simulink model "mainPacemakerUART"  (R2022b)
settings: Solver=FixedStepAuto  StartTime=0.0  StopTime=10.0  FixedStep=1e-3  RelTol=1e-3  EnableMultiTasking=on
undefined symbols (not defined in the file): A0, A1, D0, D1, D10, D11, D12, D13, D2, D3, D4, D5, D6, D7, D8, D9, PTA0, PTA1, PTA2, PTB2, PTB23, PTB3, PTB9, PTC16, PTC17, PTC2, PTC3, PTC4, PTD0, PTD1, PTD2, PTD3
libraries: frdmk64flib x19, etargetslib x10, simulink x2, dspstat3 x1
settings Model: ExtModeTrigDuration=5  Creator=christyjoseph-anton  LastModifiedBy=nickg
settings SolverCC: AlgebraicLoopSolver=TrustRegion
settings OptimizationCC: EnhancedBackFolding=on  PassReuseOutputArgsAs=Individual arguments  ZeroExternalMemoryAtStartup=off  ZeroInternalMemoryAtStartup=off  MaxStackSize=64  OptimizeBlockOrder=speed  DifferentSizesBufferReuse=on  OptimizationCustomize=off  EfficientTunableParamExpr=on
settings DebuggingCC: ParameterTunabilityLossMsg=error  UnconnectedInputMsg=warning  UnconnectedOutputMsg=warning  UnconnectedLineMsg=warning  SFMachineParentedDataDiag=warning
settings HardwareCC: ProdBitPerPointer=32  ProdBitPerSizeT=32  ProdBitPerPtrDiffT=32  ProdLargestAtomicInteger=Long  ProdLargestAtomicFloat=Double  ProdWordSize=32  ProdHWDeviceType=ARM Compatible->ARM Cortex
settings ModelReferenceCC: EnableRefExpFcnMdlSchedulingChecks=on
settings SFSimCC: MATLABDynamicMemAlloc=off
settings RTWCC: Description=Embedded Coder  SystemTargetFile=ert.tlc  HardwareBoard=NXP FRDM-K64F  TLCOptions="-aInlineSetEventsForThisBaseRateFcn=TLC_FALSE -aSuppressMultiTaskScheduler=TLC_FALSE  -aRateBasedStepFcn=0"  TemplateMakefile=ert_default_tmf  Toolchain=GNU Tools for ARM Embedded Processors  DLArmComputeVersion=19.05
settings CodeAppCC: ForceParamTrailComments=on  IgnoreCustomStorageClasses=off  OperatorAnnotations=on  SimulinkDataObjDesc=on  SFDataObjDesc=on  InsertBlockDesc=on
settings ERTTargetCC: ExtModeTransport=4  ExtModeMexFile=sendToCommService

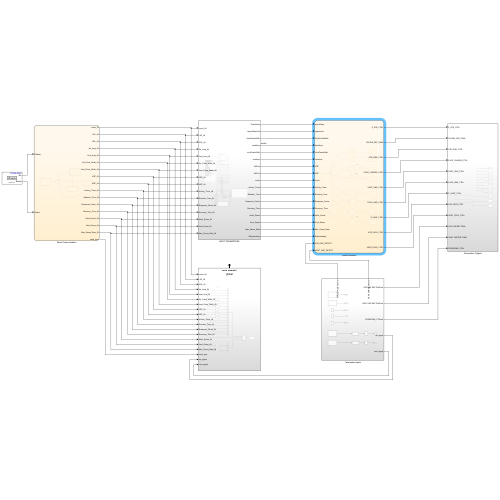
[thumbnail: Simulink's stored preview of the top-level diagram]
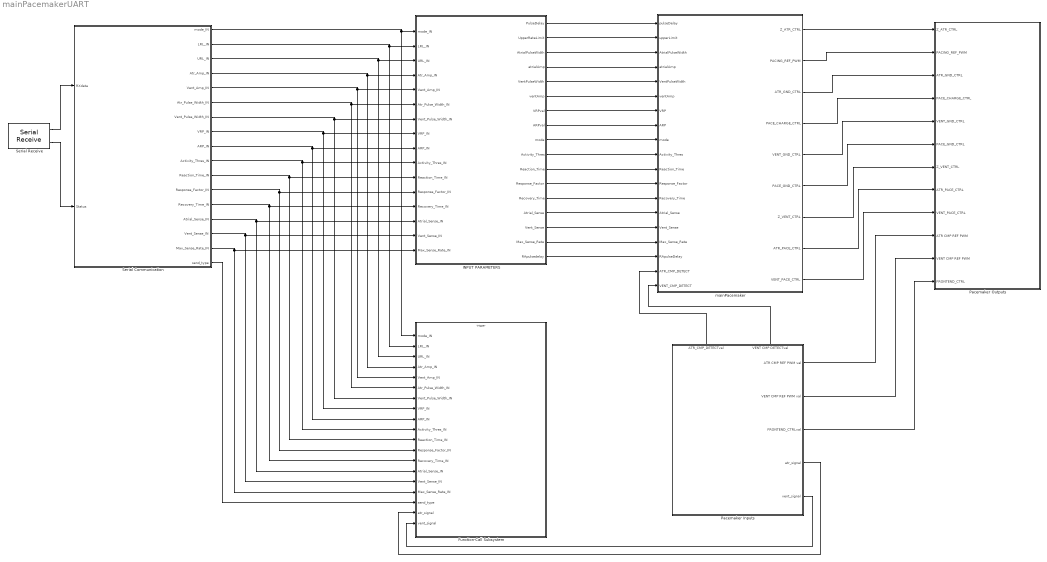
== system mainPacemakerUART ==
  Function-Call Subsystem : Subsystem  TreatAsAtomicUnit=on
  INPUT PARAMETERS : Subsystem
  Pacemaker Inputs : Subsystem
      settings: PortSchema="{\"entries\":[{\"content\":{\"sides\":[{\"content\":{\"connectorIds\":[]},\"type\":\"ConnectorPlacement.EquallySpacedRectSide\",\"uuid\":\"669aed97-6afe-41f5-9681-72417bc28ad7\"},{\"content\":{\"connectorIds\":[\"Out1\",\"Out2\",\"Out3\",\"Out4\",\"Out5\"],\"side\":\"RIGHT\"},\"type\":\"ConnectorPlacement.EquallySpacedRectSide\",\"uuid\":\"4d5229ba-5f7f-4491-b5d3-5b44c05a4562\"},{\"content\":{\"connectorIds\":[\"Out6\",\"Out7\"],\"side\":\"TOP\"},\"type\":\"ConnectorPlacement.EquallySpacedRectSide\",\"uuid\":\"a8fa4d81-6f15-4faa-ada6-82cdebea0c9a\"},{\"content\":{\"connectorIds\":[],\"side\":\"HIDDEN\"},\"type\":\"ConnectorPlacement.EquallySpacedRectSide\",\"uuid\":\"2be4ddd2-f58e-4c63-9a31-28b31fed5141\"}]},\"type\":\"ConnectorPlacement.EquallySpacedConnector\",\"uuid\":\"3d10de13-acf3-4b06-8558-a802ff7a980e\"}],\"packageUris\":[\"http://schema.mathworks.com/mf0/Connector/R2020b\"],\"version\":\"1.0\"}"
  Pacemaker Outputs : Subsystem
  Serial Communication : Stateflow chart  TreatAsAtomicUnit=on
      settings: PortSchema="{\"entries\":[{\"content\":{\"sides\":[{\"content\":{\"connectorIds\":[\"In1\",\"In2\"]},\"type\":\"ConnectorPlacement.EquallySpacedRectSide\",\"uuid\":\"155cda33-ed32-4503-9511-04db69497ed1\"},{\"content\":{\"connectorIds\":[\"Out1\",\"Out2\",\"Out3\",\"Out4\",\"Out5\",\"Out6\",\"Out7\",\"Out8\",\"Out9\",\"Out10\",\"Out11\",\"Out12\",\"Out13\",\"Out15\",\"Out16\",\"Out17\",\"Out14\"],\"side\":\"RIGHT\"},\"type\":\"ConnectorPlacement.EquallySpacedRectSide\",\"uuid\":\"03ebeb28-7a83-492d-8c6c-4e2462ffa620\"},{\"content\":{\"connectorIds\":[],\"side\":\"TOP\"},\"type\":\"ConnectorPlacement.EquallySpacedRectSide\",\"uuid\":\"df4d072d-cc91-443f-87bb-f397160e1321\"},{\"content\":{\"connectorIds\":[],\"side\":\"HIDDEN\"},\"type\":\"ConnectorPlacement.EquallySpacedRectSide\",\"uuid\":\"7e82692c-c04b-4422-948f-81d628cdafb4\"}]},\"type\":\"ConnectorPlacement.EquallySpacedConnector\",\"uuid\":\"d94360bd-ed44-4ec4-9498-3e1b8fe58b8b\"}],\"packageUris\":[\"http://schema.mathworks.com/mf0/Connector/R2020b\"],\"version\":\"1.0\"}"
  Serial Receive : frdmk64flib/Serial Receive  SCIModule=0  Baudrate=uint32(9600)  Parity=None  StopBits=1  HardwareFlowControl=None  ByteOrder=LittleEndian  DataType=uint8  DataLength=74  BlockingMode=off  OutputStatus=on  SampleTime=-1
  mainPacemaker : Stateflow chart  TreatAsAtomicUnit=on
      settings: PortSchema="{\"entries\":[{\"content\":{\"sides\":[{\"content\":{\"connectorIds\":[\"In1\",\"In2\",\"In3\",\"In4\",\"In6\",\"In7\",\"In8\",\"In9\",\"In5\",\"In10\",\"In11\",\"In12\",\"In13\",\"In14\",\"In15\",\"In18\",\"In17\",\"In16\",\"In19\"]},\"type\":\"ConnectorPlacement.EquallySpacedRectSide\",\"uuid\":\"201ff05f-9430-4aaf-95e3-1c7ad2916a7e\"},{\"content\":{\"connectorIds\":[\"Out1\",\"Out2\",\"Out3\",\"Out4\",\"Out5\",\"Out6\",\"Out7\",\"Out8\",\"Out9\"],\"side\":\"RIGHT\"},\"type\":\"ConnectorPlacement.EquallySpacedRectSide\",\"uuid\":\"5d74b1aa-6a43-4298-b365-ae775337f59f\"},{\"content\":{\"connectorIds\":[],\"side\":\"TOP\"},\"type\":\"ConnectorPlacement.EquallySpacedRectSide\",\"uuid\":\"2dd794d3-9ac6-4b1a-b21d-1675ed402b7f\"},{\"content\":{\"connectorIds\":[],\"side\":\"HIDDEN\"},\"type\":\"ConnectorPlacement.EquallySpacedRectSide\",\"uuid\":\"1f2ef5a6-ce50-482f-afd9-c477b13c6922\"}]},\"type\":\"ConnectorPlacement.EquallySpacedConnector\",\"uuid\":\"6e887b8a-81a7-4209-ac77-3100cf09278d\"}],\"packageUris\":[\"http://schema.mathworks.com/mf0/Connector/R2020b\"],\"version\":\"1.0\"}"
  wires:
  INPUT PARAMETERS/3(AtrialPulseWidth) -> mainPacemaker/3(AtrialPulseWidth)
  INPUT PARAMETERS/4(atrialAmp) -> mainPacemaker/4(atrialAmp)
  INPUT PARAMETERS/1(PulseDelay) -> mainPacemaker/1(pulseDelay)
  INPUT PARAMETERS/2(UpperRateLimit) -> mainPacemaker/2(upperLimit)
  INPUT PARAMETERS/5(VentPulseWidth) -> mainPacemaker/6(VentPulseWidth)
  INPUT PARAMETERS/6(ventAmp) -> mainPacemaker/7(ventAmp)
  INPUT PARAMETERS/7(VRPval) -> mainPacemaker/8(VRP)
  INPUT PARAMETERS/8(ARPval) -> mainPacemaker/9(ARP)
  Pacemaker Inputs/6(ATR_CMP_DETECTval) -> mainPacemaker/16(ATR_CMP_DETECT)
  Pacemaker Inputs/7(VENT CMP DETECTval) -> mainPacemaker/19(VENT_CMP_DETECT)
  mainPacemaker/1(Z_ATR_CTRL) -> Pacemaker Outputs/1(Z_ATR_CTRL)
  mainPacemaker/2(PACING_REF_PWM) -> Pacemaker Outputs/2(PACING_REF_PWM)
  mainPacemaker/3(ATR_GND_CTRL) -> Pacemaker Outputs/3(ATR_GND_CTRL)
  mainPacemaker/4(PACE_CHARGE_CTRL) -> Pacemaker Outputs/4(PACE_CHARGE_CTRL)
  mainPacemaker/5(VENT_GND_CTRL) -> Pacemaker Outputs/5(VENT_GND_CTRL)
  mainPacemaker/6(PACE_GND_CTRL) -> Pacemaker Outputs/6(PACE_GND_CTRL)
  mainPacemaker/7(Z_VENT_CTRL) -> Pacemaker Outputs/7(Z_VENT_CTRL)
  mainPacemaker/8(ATR_PACE_CTRL) -> Pacemaker Outputs/8(ATR_PACE_CTRL)
  mainPacemaker/9(VENT_PACE_CTRL) -> Pacemaker Outputs/9(VENT_PACE_CTRL)
  Pacemaker Inputs/1(ATR CMP REF PWM val) -> Pacemaker Outputs/10(ATR CMP REF PWM)
  Pacemaker Inputs/2(VENT CMP REF PWM val) -> Pacemaker Outputs/11(VENT CMP REF PWM)
  Pacemaker Inputs/3(FRONTEND_CTRLval) -> Pacemaker Outputs/12(FRONTEND_CTRL)
  INPUT PARAMETERS/9(mode) -> mainPacemaker/5(mode)
  Serial Communication/1(mode_IN) -> Function-Call Subsystem/1(mode_IN), INPUT PARAMETERS/1(mode_IN)
  Serial Communication/2(LRL_IN) -> Function-Call Subsystem/2(LRL_IN), INPUT PARAMETERS/2(LRL_IN)
  Serial Communication/3(URL_IN) -> Function-Call Subsystem/3(URL_IN), INPUT PARAMETERS/3(URL_IN)
  Serial Communication/4(Atr_Amp_IN) -> Function-Call Subsystem/4(Atr_Amp_IN), INPUT PARAMETERS/4(Atr_Amp_IN)
  Serial Communication/5(Vent_Amp_IN) -> Function-Call Subsystem/5(Vent_Amp_IN), INPUT PARAMETERS/5(Vent_Amp_IN)
  Serial Communication/6(Atr_Pulse_Width_IN) -> Function-Call Subsystem/6(Atr_Pulse_Width_IN), INPUT PARAMETERS/6(Atr_Pulse_Width_IN)
  Serial Communication/7(Vent_Pulse_Width_IN) -> Function-Call Subsystem/7(Vent_Pulse_Width_IN), INPUT PARAMETERS/7(Vent_Pulse_Width_IN)
  Serial Communication/8(VRP_IN) -> Function-Call Subsystem/8(VRP_IN), INPUT PARAMETERS/8(VRP_IN)
  Serial Communication/9(ARP_IN) -> Function-Call Subsystem/9(ARP_IN), INPUT PARAMETERS/9(ARP_IN)
  Serial Receive/2 -> Serial Communication/2(Status)
  Serial Receive/1 -> Serial Communication/1(RXdata)
  Serial Communication/10(Activity_Thres_IN) -> INPUT PARAMETERS/10(Activity_Thres_IN), Function-Call Subsystem/10(Activity_Thres_IN)
  Serial Communication/11(Reaction_Time_IN) -> Function-Call Subsystem/11(Reaction_Time_IN), INPUT PARAMETERS/11(Reaction_Time_IN)
  Serial Communication/12(Response_Factor_IN) -> Function-Call Subsystem/12(Response_Factor_IN), INPUT PARAMETERS/12(Response_Factor_IN)
  Serial Communication/13(Recovery_Time_IN) -> Function-Call Subsystem/13(Recovery_Time_IN), INPUT PARAMETERS/13(Recovery_Time_IN)
  INPUT PARAMETERS/10(Activity_Thres) -> mainPacemaker/10(Activity_Thres)
  INPUT PARAMETERS/11(Reaction_Time) -> mainPacemaker/11(Reaction_Time)
  INPUT PARAMETERS/12(Response_Factor) -> mainPacemaker/12(Response_Factor)
  INPUT PARAMETERS/13(Recovery_Time) -> mainPacemaker/13(Recovery_Time)
  Serial Communication/14(send_type) -> Function-Call Subsystem/17(send_type)
  Pacemaker Inputs/4(atr_signal) -> Function-Call Subsystem/18(atr_signal)
  Pacemaker Inputs/5(vent_signal) -> Function-Call Subsystem/19(vent_signal)
  INPUT PARAMETERS/14(Atrial_Sense) -> mainPacemaker/14(Atrial_Sense)
  INPUT PARAMETERS/15(Vent_Sense) -> mainPacemaker/15(Vent_Sense)
  INPUT PARAMETERS/16(Max_Sense_Rate) -> mainPacemaker/18(Max_Sense_Rate)
  Serial Communication/15(Atrial_Sense_IN) -> INPUT PARAMETERS/14(Atrial_Sense_IN), Function-Call Subsystem/14(Atrial_Sense_IN)
  Serial Communication/16(Vent_Sense_IN) -> INPUT PARAMETERS/15(Vent_Sense_IN), Function-Call Subsystem/15(Vent_Sense_IN)
  Serial Communication/17(Max_Sense_Rate_IN) -> INPUT PARAMETERS/16(Max_Sense_Rate_IN), Function-Call Subsystem/16(Max_Sense_Rate_IN)
  INPUT PARAMETERS/17(RApulsedelay) -> mainPacemaker/17(RApulseDelay)

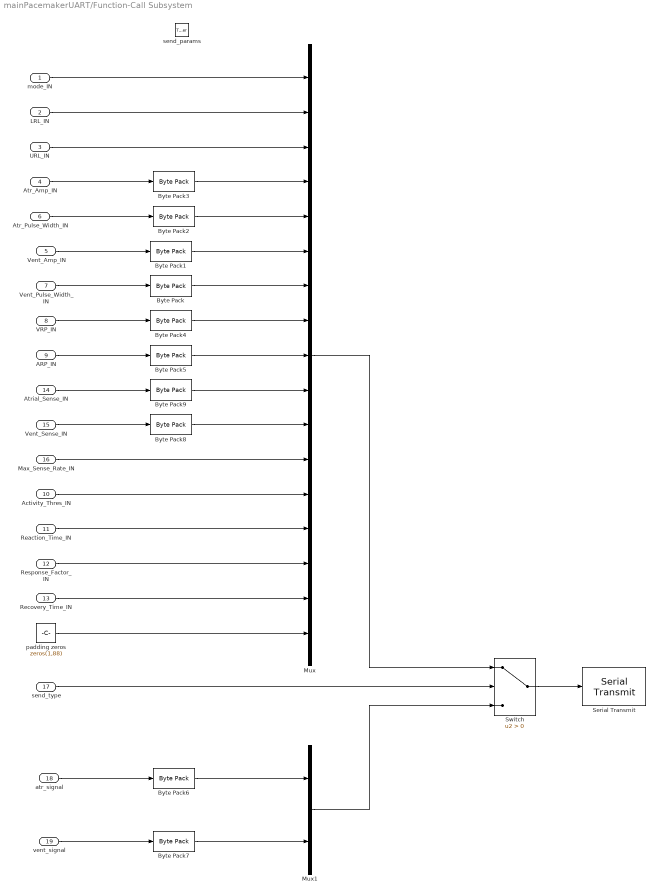
== system mainPacemakerUART/Function-Call Subsystem ==
  mode_IN : Inport
  LRL_IN : Inport  Port=2
  URL_IN : Inport  Port=3
  Atr_Amp_IN : Inport  Port=4
  Vent_Amp_IN : Inport  Port=5
  Atr_Pulse_Width_IN : Inport  Port=6
  Vent_Pulse_Width_IN : Inport  Port=7
  VRP_IN : Inport  Port=8
  ARP_IN : Inport  Port=9
  Activity_Thres_IN : Inport  Port=10
  Reaction_Time_IN : Inport  Port=11
  Response_Factor_IN : Inport  Port=12
  Recovery_Time_IN : Inport  Port=13
  Atrial_Sense_IN : Inport  Port=14
  Vent_Sense_IN : Inport  Port=15
  Max_Sense_Rate_IN : Inport  Port=16
  send_type : Inport  Port=17
  atr_signal : Inport  Port=18
  vent_signal : Inport  Port=19
  send_params : TriggerPort  TriggerType=function-call  IsSimulinkFunction=on  FunctionName=send_params  VariantControl=Variant
  Byte Pack{,1..9} (10 alike) : etargetslib/Byte Pack  datatypes={'double'}  byteAlign=1
  Mux : Mux  Inputs=17
  Mux1 : Mux  Inputs=2
  Serial Transmit : frdmk64flib/Serial Transmit  SCIModule=0  Baudrate=uint32(9600)  Parity=None  StopBits=1  HardwareFlowControl=None  ByteOrder=LittleEndian  BlockingMode=on  OutputStatus=off
  Switch : Switch  Criteria=u2 > Threshold  SaturateOnIntegerOverflow=off  InputSameDT=off
  padding zeros : Constant  Value=zeros(1,88)  OutDataTypeStr=uint8
  wires:
  mode_IN/1 -> Mux/1
  LRL_IN/1 -> Mux/2
  URL_IN/1 -> Mux/3
  Atr_Amp_IN/1 -> Byte Pack3/1
  Atr_Pulse_Width_IN/1 -> Byte Pack2/1
  Vent_Amp_IN/1 -> Byte Pack1/1
  Vent_Pulse_Width_IN/1 -> Byte Pack/1
  VRP_IN/1 -> Byte Pack4/1
  ARP_IN/1 -> Byte Pack5/1
  Byte Pack/1 -> Mux/7
  Byte Pack1/1 -> Mux/6
  Byte Pack3/1 -> Mux/4
  Byte Pack2/1 -> Mux/5
  Byte Pack4/1 -> Mux/8
  Byte Pack5/1 -> Mux/9
  Switch/1 -> Serial Transmit/1
  Mux/1 -> Switch/1
  send_type/1 -> Switch/2
  Mux1/1 -> Switch/3
  atr_signal/1 -> Byte Pack6/1
  Byte Pack6/1 -> Mux1/1
  vent_signal/1 -> Byte Pack7/1
  Byte Pack7/1 -> Mux1/2
  padding zeros/1 -> Mux/17
  Atrial_Sense_IN/1 -> Byte Pack9/1
  Vent_Sense_IN/1 -> Byte Pack8/1
  Activity_Thres_IN/1 -> Mux/13
  Reaction_Time_IN/1 -> Mux/14
  Response_Factor_IN/1 -> Mux/15
  Recovery_Time_IN/1 -> Mux/16
  Byte Pack8/1 -> Mux/11
  Max_Sense_Rate_IN/1 -> Mux/12
  Byte Pack9/1 -> Mux/10

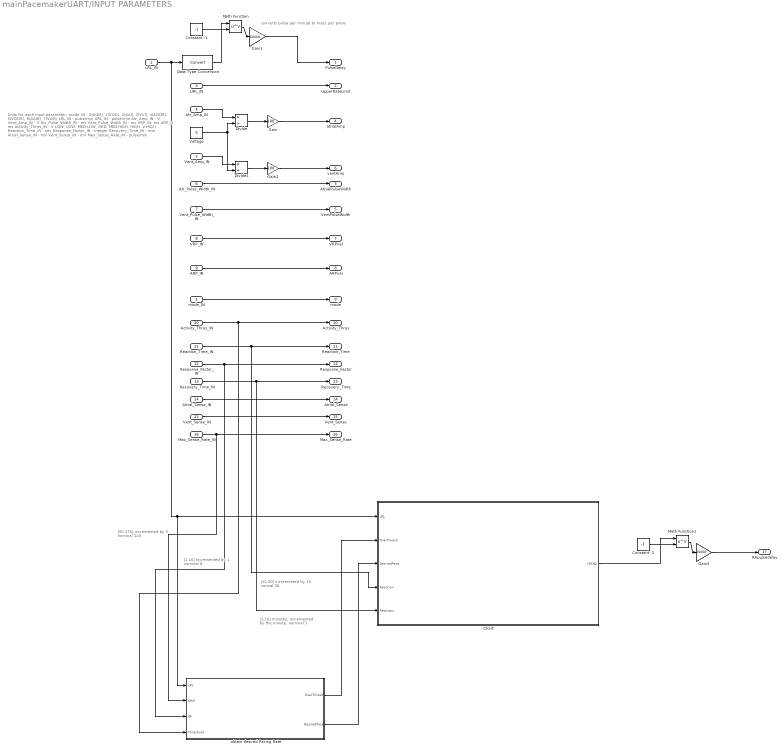
== system mainPacemakerUART/INPUT PARAMETERS ==
  note: Units for each input parameter:
      | mode_IN - 0(AOO), 1(VOO), 2(AAI), 3(VVI), 4(AOOR), 5(VOOR), 6(AAIR), 7(VVIR)
      |
      | LRL_IN - pulse/min
      |
      | URL_IN - pulse/min
      |
      | Atr_Amp_IN - V
      |
      | Vent_Amp_IN - V
      |
      | Atr_Pulse_Width_IN - ms
      |
      | Vent_Pulse_Width_IN - ms
      |
      | VRP_IN- ms ARP_N - ms
      |
      | Activity_Thres_IN - V-LOW, LOW, MED-LOW, MED, MED-HIGH, HIGH, V-HIGH
      |
      | Reaction_Time_IN - sec
      |
      | Response_Factor_IN - integer
      |
      | Recovery_Time_IN - min Atrial_Sense_IN - mV
      |
      | Vent_Sense_IN - mV
      |
      | Max_Sense_Rate_IN - pulse/min
  note: converts pulse per minute to msec per pulse
  note: [2,16] minutes, incremented by the minute, nominal 5
  note: [10,50] incremented by 10 nomial 30
  note: [50,175] incremented by 5 nominal 120
  note: [1,16] incremented by 1, nominal 8
  mode_IN : Inport
  LRL_IN : Inport  Port=2
  URL_IN : Inport  Port=3
  Atr_Amp_IN : Inport  Port=4
  Vent_Amp_IN : Inport  Port=5
  Atr_Pulse_Width_IN : Inport  Port=6
  Vent_Pulse_Width_IN : Inport  Port=7
  VRP_IN : Inport  Port=8
  ARP_IN : Inport  Port=9
  Activity_Thres_IN : Inport  Port=10
  Reaction_Time_IN : Inport  Port=11
  Response_Factor_IN : Inport  Port=12
  Recovery_Time_IN : Inport  Port=13
  Atrial_Sense_IN : Inport  Port=14
  Vent_Sense_IN : Inport  Port=15
  Max_Sense_Rate_IN : Inport  Port=16
  Chart : Stateflow chart  TreatAsAtomicUnit=on
  Constant -1 : Constant  Value=-1
  Constant -2 : Constant  Value=-1
  Data Type Conversion : DataTypeConversion  SaturateOnIntegerOverflow=off  RndMeth=Floor
  Divide : Product  Inputs=*/
  Divide1 : Product  Inputs=*/
  Gain : Gain  Gain=100
  Gain1 : Gain  Gain=60000
  Gain2 : Gain  Gain=100
  Gain3 : Gain  Gain=60000
  Math Function : Math  Operator=pow
  Math Function1 : Math  Operator=pow
  Voltage : Constant  Value=5
  obtain desired Pacing Rate : Subsystem
  PulseDelay : Outport
  UpperRateLimit : Outport  Port=2
  AtrialPulseWidth : Outport  Port=3
  atrialAmp : Outport  Port=4  OutDataTypeStr=double
  VentPulseWidth : Outport  Port=5
  ventAmp : Outport  Port=6
  VRPval : Outport  Port=7
  ARPval : Outport  Port=8
  mode : Outport  Port=9
  Activity_Thres : Outport  Port=10
  Reaction_Time : Outport  Port=11
  Response_Factor : Outport  Port=12
  Recovery_Time : Outport  Port=13
  Atrial_Sense : Outport  Port=14
  Vent_Sense : Outport  Port=15
  Max_Sense_Rate : Outport  Port=16
  RApulsedelay : Outport  Port=17
  wires:
  Gain/1 -> atrialAmp/1
  Constant -1/1 -> Math Function/2
  Math Function/1 -> Gain1/1
  Atr_Amp_IN/1 -> Divide/1
  Gain1/1 -> PulseDelay/1
  URL_IN/1 -> UpperRateLimit/1
  Atr_Pulse_Width_IN/1 -> AtrialPulseWidth/1
  Divide/1 -> Gain/1
  Voltage/1 -> Divide1/2, Divide/2
  Gain2/1 -> ventAmp/1
  Vent_Amp_IN/1 -> Divide1/1
  Divide1/1 -> Gain2/1
  Vent_Pulse_Width_IN/1 -> VentPulseWidth/1
  VRP_IN/1 -> VRPval/1
  ARP_IN/1 -> ARPval/1
  mode_IN/1 -> mode/1
  Data Type Conversion/1 -> Math Function/1
  Vent_Sense_IN/1 -> Vent_Sense/1
  Atrial_Sense_IN/1 -> Atrial_Sense/1
  Recovery_Time_IN/1 -> Chart/5(Recovery), Recovery_Time/1
  Activity_Thres_IN/1 -> obtain desired Pacing Rate/4(Threshold), Activity_Thres/1
  Reaction_Time_IN/1 -> Chart/4(Reaction), Reaction_Time/1
  obtain desired Pacing Rate/2(DesiredPace) -> Chart/3(DesiredPace)
  obtain desired Pacing Rate/1(OverThresh) -> Chart/2(OverThresh)
  Response_Factor_IN/1 -> Response_Factor/1, obtain desired Pacing Rate/3(RF)
  LRL_IN/1 -> Chart/1(LRL), obtain desired Pacing Rate/1(LRL), Data Type Conversion/1
  Max_Sense_Rate_IN/1 -> obtain desired Pacing Rate/2(MSR), Max_Sense_Rate/1
  Math Function1/1 -> Gain3/1
  Chart/1(LRLRA) -> Math Function1/1
  Constant -2/1 -> Math Function1/2
  Gain3/1 -> RApulsedelay/1

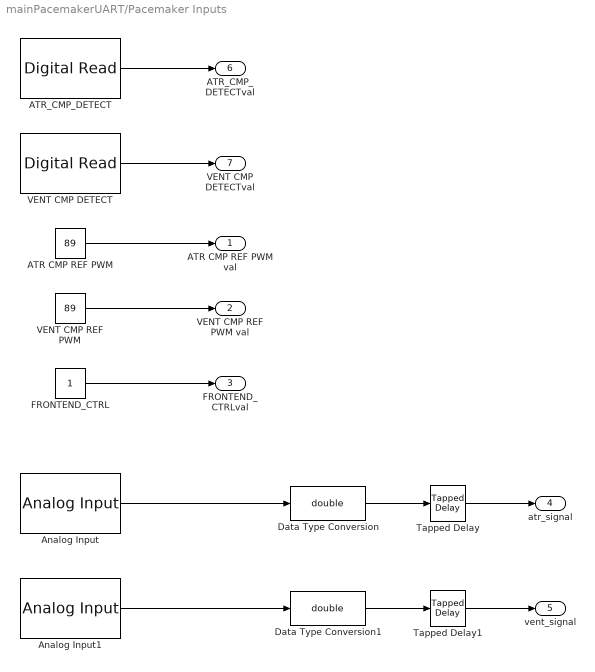
== system mainPacemakerUART/Pacemaker Inputs ==
  ATR CMP REF PWM : Constant  Value=89
  ATR_CMP_DETECT : frdmk64flib/Digital Read  Whichpin=PTC16 (D0)  SampleTime=-1
  Analog Input : frdmk64flib/Analog Input  Whichpin=PTB2 (A0)  SampleTime=-1
  Analog Input1 : frdmk64flib/Analog Input  Whichpin=PTB3 (A1)  SampleTime=-1
  Data Type Conversion : DataTypeConversion  OutDataTypeStr=double  SaturateOnIntegerOverflow=off  RndMeth=Floor
  Data Type Conversion1 : DataTypeConversion  OutDataTypeStr=double  SaturateOnIntegerOverflow=off  RndMeth=Floor
  FRONTEND_CTRL : Constant
  Tapped Delay : simulink/Discrete/Tapped Delay  vinit=1  samptime=0.002  NumDelays=10  DelayOrder=Oldest  includeCurrent=off
  Tapped Delay1 : simulink/Discrete/Tapped Delay  vinit=0.0  samptime=0.002  NumDelays=10  DelayOrder=Oldest  includeCurrent=off
  VENT CMP DETECT : frdmk64flib/Digital Read  Whichpin=PTC17 (D1)  SampleTime=-1
  VENT CMP REF PWM : Constant  Value=89
  ATR CMP REF PWM val : Outport
  VENT CMP REF PWM val : Outport  Port=2
  FRONTEND_CTRLval : Outport  Port=3
  atr_signal : Outport  Port=4
  vent_signal : Outport  Port=5
  ATR_CMP_DETECTval : Outport  Port=6
  VENT CMP DETECTval : Outport  Port=7
  wires:
  VENT CMP DETECT/1 -> VENT CMP DETECTval/1
  VENT CMP REF PWM/1 -> VENT CMP REF PWM val/1
  ATR_CMP_DETECT/1 -> ATR_CMP_DETECTval/1
  ATR CMP REF PWM/1 -> ATR CMP REF PWM val/1
  FRONTEND_CTRL/1 -> FRONTEND_CTRLval/1
  Analog Input/1 -> Data Type Conversion/1
  Data Type Conversion/1 -> Tapped Delay/1
  Analog Input1/1 -> Data Type Conversion1/1
  Data Type Conversion1/1 -> Tapped Delay1/1
  Tapped Delay/1 -> atr_signal/1
  Tapped Delay1/1 -> vent_signal/1

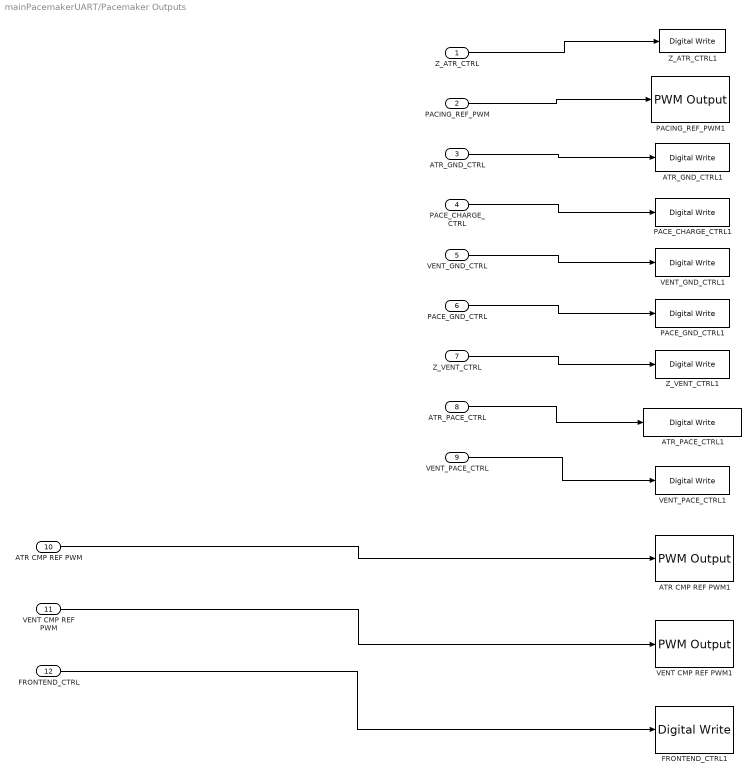
== system mainPacemakerUART/Pacemaker Outputs ==
  Z_ATR_CTRL : Inport
  PACING_REF_PWM : Inport  Port=2
  ATR_GND_CTRL : Inport  Port=3
  PACE_CHARGE_CTRL : Inport  Port=4
  VENT_GND_CTRL : Inport  Port=5
  PACE_GND_CTRL : Inport  Port=6
  Z_VENT_CTRL : Inport  Port=7
  ATR_PACE_CTRL : Inport  Port=8
  VENT_PACE_CTRL : Inport  Port=9
  ATR CMP REF PWM : Inport  Port=10
  VENT CMP REF PWM : Inport  Port=11
  FRONTEND_CTRL : Inport  Port=12
  ATR CMP REF PWM1 : frdmk64flib/PWM Output  Whichpin=PTC2 (D6)  InitialFrequency=2000  InitialDutyCycle=0
  ATR_GND_CTRL1 : frdmk64flib/Digital Write  Whichpin=PTD2 (D11)
  ATR_PACE_CTRL1 : frdmk64flib/Digital Write  Whichpin=PTA0 (D8)
  FRONTEND_CTRL1 : frdmk64flib/Digital Write  Whichpin=PTD1 (D13)
  PACE_CHARGE_CTRL1 : frdmk64flib/Digital Write  Whichpin=PTB9 (D2)
  PACE_GND_CTRL1 : frdmk64flib/Digital Write  Whichpin=PTD0 (D10)
  PACING_REF_PWM1 : frdmk64flib/PWM Output  Whichpin=PTA2 (D5)  InitialFrequency=2000  InitialDutyCycle=50
  VENT CMP REF PWM1 : frdmk64flib/PWM Output  Whichpin=PTA1 (D3)  InitialFrequency=2000  InitialDutyCycle=0
  VENT_GND_CTRL1 : frdmk64flib/Digital Write  Whichpin=PTD3 (D12)
  VENT_PACE_CTRL1 : frdmk64flib/Digital Write  Whichpin=PTC4 (D9)
  Z_ATR_CTRL1 : frdmk64flib/Digital Write  Whichpin=PTB23 (D4)
  "Z_VENT_CTRL1 " : frdmk64flib/Digital Write  Whichpin=PTC3 (D7)
  wires:
  ATR_PACE_CTRL/1 -> ATR_PACE_CTRL1/1
  ATR CMP REF PWM/1 -> ATR CMP REF PWM1/1
  PACING_REF_PWM/1 -> PACING_REF_PWM1/1
  VENT_GND_CTRL/1 -> VENT_GND_CTRL1/1
  VENT CMP REF PWM/1 -> VENT CMP REF PWM1/1
  VENT_PACE_CTRL/1 -> VENT_PACE_CTRL1/1
  PACE_CHARGE_CTRL/1 -> PACE_CHARGE_CTRL1/1
  Z_VENT_CTRL/1 -> "Z_VENT_CTRL1 "/1
  Z_ATR_CTRL/1 -> Z_ATR_CTRL1/1
  ATR_GND_CTRL/1 -> ATR_GND_CTRL1/1
  FRONTEND_CTRL/1 -> FRONTEND_CTRL1/1
  PACE_GND_CTRL/1 -> PACE_GND_CTRL1/1

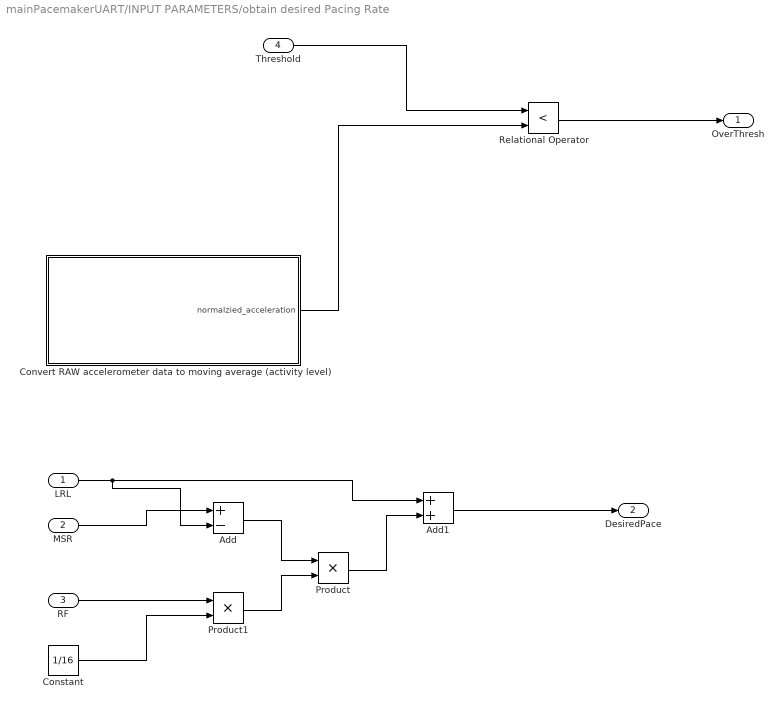
== system mainPacemakerUART/INPUT PARAMETERS/obtain desired Pacing Rate ==
  LRL : Inport
  MSR : Inport  Port=2
  RF : Inport  Port=3
  Threshold : Inport  Port=4
  Add : Sum  Inputs=+-
  Add1 : Sum
  Constant : Constant  Value=1/16
  Convert RAW accelerometer data to moving average (activity level) : Subsystem
  Product : Product
  Product1 : Product
  Relational Operator : RelationalOperator  Operator=<  OutDataTypeStr=boolean  RndMeth=Simplest  InputSameDT=off
  OverThresh : Outport
  DesiredPace : Outport  Port=2
  wires:
  MSR/1 -> Add/1
  LRL/1 -> Add/2, Add1/1
  Add/1 -> Product/1
  Product/1 -> Add1/2
  Threshold/1 -> Relational Operator/1
  Add1/1 -> DesiredPace/1
  Relational Operator/1 -> OverThresh/1
  Convert RAW accelerometer data to moving average (activity level)/1(normalzied_acceleration) -> Relational Operator/2
  RF/1 -> Product1/1
  Constant/1 -> Product1/2
  Product1/1 -> Product/2

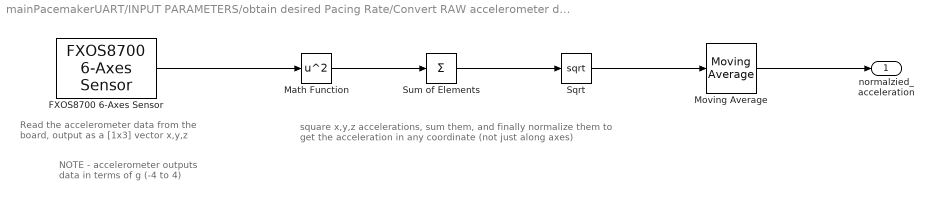
== system mainPacemakerUART/INPUT PARAMETERS/obtain desired Pacing Rate/Convert RAW accelerometer data to moving average (activity level) ==
  note: NOTE - accelerometer outputs data in terms of g (-4 to 4)
  note: square x,y,z accelerations, sum them, and finally normalize them to get the acceleration in any coordinate (not just along axes)
  note: Read the accelerometer data from the board, output as a [1x3] vector x,y,z
  FXOS8700 6-Axes Sensor : frdmk64flib/FXOS8700 6-Axes Sensor  Activesensor=Accelerometer only  ODR=800Hz  HybridODR=400Hz  Accelfullrange=-4g to +4g  SampleTime=-1
  Math Function : Math  Operator=square
  Moving Average : dspstat3/Moving Average  Method=Sliding window  ForgettingFactorPort=off  SpecifyWindowLength=on  WindowLength=4  OverlapLength=3  AllowArbitraryInputLength=off  ForgettingFactor=0.9  SimulateUsing=Code generation
  Sqrt : Sqrt
  Sum of Elements : Sum  Inputs=+
  normalzied_acceleration : Outport
  wires:
  Sum of Elements/1 -> Sqrt/1
  Sqrt/1 -> Moving Average/1
  Moving Average/1 -> normalzied_acceleration/1
  FXOS8700 6-Axes Sensor/1 -> Math Function/1
  Math Function/1 -> Sum of Elements/1

== stateflow chart mainPacemakerUART/Serial Communication ==
  settings: executeAtInitialization=1
  state SET_PARM
    entry:
    mode_IN=RXdata(3); %1B
    LRL_IN=RXdata(4); %1B
    URL_IN=RXdata(5); %1B
    Atr_Amp_IN=typecast(RXdata(6:13),'double'); %8B
    Atr_Pulse_Width_IN=typecast(RXdata(14:21),'double'); %8B
    Vent_Amp_IN=typecast(RXdata(22:29),'double') %8B
    Vent_Pulse_Width_IN=typecast(RXdata(30:37),'double'); %8B
    VRP_IN=typecast(RXdata(38:45),'double'); %8B
    ARP_IN=typecast(RXdata(46:53),'double'); %8B
    Atrial_Sense_IN=typecast(RXdata(54:61),'double'); %8B
    Vent_Sense_IN=typecast(RXdata(62:69),'double'); %8B
    Max_Sense_Rate_IN=RXdata(70); %1B
    Activity_Thres_IN=RXdata(71); %1B
    Reaction_Time_IN=RXdata(72); %1B
    Response_Factor_IN=RXdata(73); %1B
    Recovery_Time_IN=RXdata(74); %1B
  state setDefault
    entry:
    mode_IN = 3;
    LRL_IN = 60;
    URL_IN = 120;
    Atr_Amp_IN = 3.3;
    Vent_Amp_IN = 3.3;
    Atr_Pulse_Width_IN = 20;
    Vent_Pulse_Width_IN = 20;
    VRP_IN=320;
    ARP_IN=250;
    Activity_Thres_IN=3;
    Reaction_Time_IN=30;
    Response_Factor_IN=8;
    Recovery_Time_IN=5;
    Atrial_Sense_IN=0.75;
    Vent_Sense_IN=2.5;
    Max_Sense_Rate_IN=120;
  state STANDBY
    %Waiting for COM
  state ECHO_PARAM
    entry:
    send_type=1; %signals send block to echo parameters
    send_params();
  state ECG_SEND
    entry:
    send_type=0; %signals send block to send  ECG data
    send_params();
  SET_PARM -> STANDBY
  (junction 11) -> SET_PARM [order 1] : [RXdata(2)==hex2dec('55')]
  (default) -> setDefault
  (junction 8) -> STANDBY [order 2]
  setDefault -> STANDBY
  STANDBY -> (junction 8) : [Status==0]
  (junction 8) -> (junction 11) [order 1] : [RXdata(1)==hex2dec('16')]
  (junction 11) -> ECHO_PARAM [order 2] : [RXdata(2)==hex2dec('22')]
  (junction 11) -> ECG_SEND [order 3] : [RXdata(2)==hex2dec('77')]
  ECHO_PARAM -> STANDBY
  ECG_SEND -> STANDBY
  data: RXdata input uint8; Status input uint8; mode_IN output uint8; LRL_IN output uint8; URL_IN output uint8; Atr_Amp_IN output double; Vent_Amp_IN output double; Atr_Pulse_Width_IN output double; Vent_Pulse_Width_IN output double; VRP_IN output double; ARP_IN output double; Activity_Thres_IN output uint8; Reaction_Time_IN output uint8; Response_Factor_IN output uint8; Recovery_Time_IN output uint8; send_type output uint8; Atrial_Sense_IN output double; Vent_Sense_IN output double; Max_Sense_Rate_IN output uint8

== stateflow chart mainPacemakerUART/INPUT PARAMETERS/Chart ==
  state IncreaseRate
    LRLRA = LRLRA + ((double(DesiredPace) - double(LRL)) / double(Reaction)) / (1000)
  state S1
    LRLRA = double(LRL)
  state HoldDesiredPace
    LRLRA = double(DesiredPace)
  state ActivityBroken [commented out]
  state DecreaseRate
    LRLRA = LRLRA - ((double(DesiredPace) - double(LRL)) / double(Recovery)) / (1000)
  IncreaseRate -> HoldDesiredPace : [LRLRA >= DesiredPace]
  S1 -> IncreaseRate : [OverThresh == 1]
  DecreaseRate -> IncreaseRate [commented out] : [OverThresh == 1]
  IncreaseRate -> ActivityBroken [commented out] : [OverThresh ~= 1]
  ActivityBroken -> IncreaseRate [commented out] : [OverThresh == 1]
  (default) -> S1
  HoldDesiredPace -> DecreaseRate : [duration(OverThresh ~= 1) > Reaction]
  DecreaseRate -> S1 : [LRLRA <= LRL]
  ActivityBroken -> DecreaseRate [commented out] : [after(5, sec)]
  data: LRL input; LRLRA output; OverThresh input; DesiredPace input; Reaction input; Recovery input

== stateflow chart mainPacemakerUART/mainPacemaker ==
  state PacingAOO
    during:
    %Discharge C22 into Atrium and charge C21
    PACE_CHARGE_CTRL = LOW
    PACE_GND_CTRL = HIGH
    ATR_PACE_CTRL = HIGH
    ATR_GND_CTRL = LOW
    Z_ATR_CTRL = LOW
    Z_VENT_CTRL = LOW
    VENT_GND_CTRL = LOW
    VENT_PACE_CTRL  = LOW
  state ChargingAOO
    during:
    %Begin Charging C22 Capacitor
    ATR_PACE_CTRL = LOW
    VENT_PACE_CTRL = LOW
    PACING_REF_PWM = atrialAmp
    PACE_CHARGE_CTRL = HIGH
    %Begin Discharging C21 Blocking Capacitor
    PACE_GND_CTRL = HIGH
    VENT_PACE_CTRL = LOW
    Z_ATR_CTRL = LOW
    Z_VENT_CTRL = LOW
    ATR_PACE_CTRL = LOW
    ATR_GND_CTRL = HIGH
    VENT_GND_CTRL = LOW
  state PacingVOO
    during:
    %Discharge C22 into Atrium and charge C21
    PACE_CHARGE_CTRL = LOW
    PACE_GND_CTRL = HIGH
    ATR_PACE_CTRL = LOW
    ATR_GND_CTRL = LOW
    Z_ATR_CTRL = LOW
    Z_VENT_CTRL = LOW
    VENT_GND_CTRL = LOW
    VENT_PACE_CTRL  = HIGH
  state ChargingVOO
    during:
    %Begin Charging C22 Capacitor
    ATR_PACE_CTRL = LOW
    VENT_PACE_CTRL = LOW
    PACING_REF_PWM = ventAmp
    PACE_CHARGE_CTRL = HIGH
    %Begin Discharging C21 Blocking Capacitor
    PACE_GND_CTRL = HIGH
    VENT_PACE_CTRL = LOW
    Z_ATR_CTRL = LOW
    Z_VENT_CTRL = LOW
    ATR_PACE_CTRL = LOW
    ATR_GND_CTRL = LOW
    VENT_GND_CTRL = HIGH
  note: if pulse is sensed from the heart outside the refractory period, cancel pulse and go back to charge state
  state waitingState
  state ChargingAAI
    during:
    %Begin Charging C22 Capacitor
    ATR_PACE_CTRL = LOW
    VENT_PACE_CTRL = LOW
    PACING_REF_PWM = atrialAmp
    PACE_CHARGE_CTRL = HIGH
    %Begin Discharging C21 Blocking Capacitor
    PACE_GND_CTRL = HIGH
    VENT_PACE_CTRL = LOW
    Z_ATR_CTRL = LOW
    Z_VENT_CTRL = LOW
    ATR_PACE_CTRL = LOW
    ATR_GND_CTRL = HIGH
    VENT_GND_CTRL = LOW
  state Sensing
  state PacingAAI
    during:
    %Discharge C22 into Atrium and charge C21
    PACE_CHARGE_CTRL = LOW
    PACE_GND_CTRL = HIGH
    ATR_PACE_CTRL = HIGH
    ATR_GND_CTRL = LOW
    Z_ATR_CTRL = LOW
    Z_VENT_CTRL = LOW
    VENT_GND_CTRL = LOW
    VENT_PACE_CTRL  = LOW
  note: ARP starts as soon as pulse is sent, so pulse width must be subtracted before detecting pulse
  note: if heart doesn't pulse, send after pulseDelay-VRP, since pulse delay is the planned pulse duration which starts from previous pulse
  note: if pulse is sensed from the heart outside the refractory period, cancel pulse and go back to charge state
  state ModeSelection
    during:
  state waitingState2
  note: pulseWidth delay must be added back as it is apart of the last cycle
  note: ARP starts as soon as pulse is sent, so pulse width must be subtracted before detecting pulse
  note: if heart doesn't pulse, send after pulseDelay-VRP, since pulse delay is the planned pulse duration which starts from previous pulse
  state PacingVVI
    during:
    %Discharge C22 into Atrium and charge C21
    PACE_CHARGE_CTRL = LOW
    PACE_GND_CTRL = HIGH
    ATR_PACE_CTRL = LOW
    ATR_GND_CTRL = LOW
    Z_ATR_CTRL = LOW
    Z_VENT_CTRL = LOW
    VENT_GND_CTRL = LOW
    VENT_PACE_CTRL  = HIGH
  state ChargingVVI
    during:
    %Begin Charging C22 Capacitor
    ATR_PACE_CTRL = LOW
    VENT_PACE_CTRL = LOW
    PACING_REF_PWM = ventAmp
    PACE_CHARGE_CTRL = HIGH
    %Begin Discharging C21 Blocking Capacitor
    PACE_GND_CTRL = HIGH
    VENT_PACE_CTRL = LOW
    Z_ATR_CTRL = LOW
    Z_VENT_CTRL = LOW
    ATR_PACE_CTRL = LOW
    ATR_GND_CTRL = LOW
    VENT_GND_CTRL = HIGH
  state Sensing2
  state PacingAOOR
    during:
    %Discharge C22 into Atrium and charge C21
    PACE_CHARGE_CTRL = LOW
    PACE_GND_CTRL = HIGH
    ATR_PACE_CTRL = HIGH
    ATR_GND_CTRL = LOW
    Z_ATR_CTRL = LOW
    Z_VENT_CTRL = LOW
    VENT_GND_CTRL = LOW
    VENT_PACE_CTRL  = LOW
  state ChargingAOOR
    during:
    %Begin Charging C22 Capacitor
    ATR_PACE_CTRL = LOW
    VENT_PACE_CTRL = LOW
    PACING_REF_PWM = atrialAmp
    PACE_CHARGE_CTRL = HIGH
    %Begin Discharging C21 Blocking Capacitor
    PACE_GND_CTRL = HIGH
    VENT_PACE_CTRL = LOW
    Z_ATR_CTRL = LOW
    Z_VENT_CTRL = LOW
    ATR_PACE_CTRL = LOW
    ATR_GND_CTRL = HIGH
    VENT_GND_CTRL = LOW
  state PacingVOOR
    during:
    %Discharge C22 into Atrium and charge C21
    PACE_CHARGE_CTRL = LOW
    PACE_GND_CTRL = HIGH
    ATR_PACE_CTRL = LOW
    ATR_GND_CTRL = LOW
    Z_ATR_CTRL = LOW
    Z_VENT_CTRL = LOW
    VENT_GND_CTRL = LOW
    VENT_PACE_CTRL  = HIGH
  state ChargingVOOR
    during:
    %Begin Charging C22 Capacitor
    ATR_PACE_CTRL = LOW
    VENT_PACE_CTRL = LOW
    PACING_REF_PWM = ventAmp
    PACE_CHARGE_CTRL = HIGH
    %Begin Discharging C21 Blocking Capacitor
    PACE_GND_CTRL = HIGH
    VENT_PACE_CTRL = LOW
    Z_ATR_CTRL = LOW
    Z_VENT_CTRL = LOW
    ATR_PACE_CTRL = LOW
    ATR_GND_CTRL = LOW
    VENT_GND_CTRL = HIGH
  note: if pulse is sensed from the heart outside the refractory period, cancel pulse and go back to charge state
  state waitingState3
  state CHARGINGAAIR
    during:
    %Begin Charging C22 Capacitor
    ATR_PACE_CTRL = LOW
    VENT_PACE_CTRL = LOW
    PACING_REF_PWM = atrialAmp
    PACE_CHARGE_CTRL = HIGH
    %Begin Discharging C21 Blocking Capacitor
    PACE_GND_CTRL = HIGH
    VENT_PACE_CTRL = LOW
    Z_ATR_CTRL = LOW
    Z_VENT_CTRL = LOW
    ATR_PACE_CTRL = LOW
    ATR_GND_CTRL = HIGH
    VENT_GND_CTRL = LOW
  state Sensing3
  state PACINGAAIR
    during:
    %Discharge C22 into Atrium and charge C21
    PACE_CHARGE_CTRL = LOW
    PACE_GND_CTRL = HIGH
    ATR_PACE_CTRL = HIGH
    ATR_GND_CTRL = LOW
    Z_ATR_CTRL = LOW
    Z_VENT_CTRL = LOW
    VENT_GND_CTRL = LOW
    VENT_PACE_CTRL  = LOW
  note: ARP starts as soon as pulse is sent, so pulse width must be subtracted before detecting pulse
  note: if heart doesn't pulse, send after pulseDelay-VRP, since pulse delay is the planned pulse duration which starts from previous pulse
  note: if pulse is sensed from the heart outside the refractory period, cancel pulse and go back to charge state
  note: pulseWidth delay must be added back as it is apart of the last cycle
  state waitingState4
  note: ARP starts as soon as pulse is sent, so pulse width must be subtracted before detecting pulse
  note: if heart doesn't pulse, send after pulseDelay-VRP, since pulse delay is the planned pulse duration which starts from previous pulse
  state PacingVVIR
    during:
    %Discharge C22 into Atrium and charge C21
    PACE_CHARGE_CTRL = LOW
    PACE_GND_CTRL = HIGH
    ATR_PACE_CTRL = LOW
    ATR_GND_CTRL = LOW
    Z_ATR_CTRL = LOW
    Z_VENT_CTRL = LOW
    VENT_GND_CTRL = LOW
    VENT_PACE_CTRL  = HIGH
  state ChargingVVIR
    during:
    %Begin Charging C22 Capacitor
    ATR_PACE_CTRL = LOW
    VENT_PACE_CTRL = LOW
    PACING_REF_PWM = ventAmp
    PACE_CHARGE_CTRL = HIGH
    %Begin Discharging C21 Blocking Capacitor
    PACE_GND_CTRL = HIGH
    VENT_PACE_CTRL = LOW
    Z_ATR_CTRL = LOW
    Z_VENT_CTRL = LOW
    ATR_PACE_CTRL = LOW
    ATR_GND_CTRL = LOW
    VENT_GND_CTRL = HIGH
  state Sensing4
  ChargingAOO -> ModeSelection [order 2] : [mode~=uint8(0)]
  PacingAOO -> ChargingAOO : after(AtrialPulseWidth,msec)
  ModeSelection -> ChargingAOO [order 1] : [mode==uint8(0)]
  ChargingAOO -> PacingAOO [order 1] : [after(pulseDelay-AtrialPulseWidth,msec)]
  ChargingVOO -> PacingVOO [order 1] : after(pulseDelay-VentPulseWidth,msec)
  ModeSelection -> ChargingVOO [order 7] : [mode==uint8(1)]
  ChargingVOO -> ModeSelection [order 2] : [mode~=uint8(1)]
  PacingVOO -> ChargingVOO : after(VentPulseWidth,msec)
  Sensing -> waitingState [order 1] : [ATR_CMP_DETECT == 1]
  waitingState -> ChargingAAI : after(AtrialPulseWidth,msec)
  ChargingAAI -> Sensing [order 1] : after(ARP-AtrialPulseWidth,msec)
  Sensing -> PacingAAI [order 2] : after((pulseDelay-AtrialPulseWidth)-(ARP-AtrialPulseWidth),msec)
  ModeSelection -> ChargingAAI [order 8] : [mode==uint8(2)]
  ChargingAAI -> ModeSelection [order 2] : [mode~=uint8(2)]
  PacingAAI -> ChargingAAI : after(AtrialPulseWidth,msec)
  (default) -> ModeSelection
  Sensing2 -> waitingState2 [order 1] : [VENT_CMP_DETECT == 1]
  waitingState2 -> ChargingVVI : after(VentPulseWidth,msec)
  ChargingVVI -> Sensing2 [order 1] : after(VRP-VentPulseWidth,msec)
  ModeSelection -> ChargingVVI [order 2] : [mode==uint8(3)]
  Sensing2 -> PacingVVI [order 2] : after((pulseDelay-VentPulseWidth)-(VRP-VentPulseWidth),msec)
  ChargingVVI -> ModeSelection [order 2] : [mode~=uint8(3)]
  PacingVVI -> ChargingVVI : after(VentPulseWidth,msec)
  ModeSelection -> ChargingAOOR [order 6] : [mode == uint8(4)]
  ChargingAOOR -> ModeSelection [order 2] : [mode ~= uint8(4)]
  PacingAOOR -> ChargingAOOR : after(AtrialPulseWidth,msec)
  ModeSelection -> ChargingVOOR [order 5] : [mode == uint8(5)]
  ChargingAOOR -> PacingAOOR [order 1] : [after(RApulseDelay-AtrialPulseWidth,msec)]
  ChargingVOOR -> ModeSelection [order 2] : [mode ~= uint8(5)]
  ChargingVOOR -> PacingVOOR [order 1] : after(RApulseDelay-VentPulseWidth,msec)
  ModeSelection -> CHARGINGAAIR [order 4] : [mode == uint8(6)]
  PacingVOOR -> ChargingVOOR : after(VentPulseWidth,msec)
  CHARGINGAAIR -> ModeSelection [order 2] : [mode ~= uint8(6)]
  Sensing3 -> waitingState3 [order 1] : [ATR_CMP_DETECT == 1]
  waitingState3 -> CHARGINGAAIR : after(AtrialPulseWidth,msec)
  ChargingVVIR -> ModeSelection [order 2] : [mode ~= uint8(7)]
  ModeSelection -> ChargingVVIR [order 3] : [mode == uint8(7)]
  CHARGINGAAIR -> Sensing3 [order 1] : after(ARP-AtrialPulseWidth,msec)
  Sensing3 -> PACINGAAIR [order 2] : after((RApulseDelay-AtrialPulseWidth)-(ARP-AtrialPulseWidth),msec)
  PACINGAAIR -> CHARGINGAAIR : after(AtrialPulseWidth,msec)
  Sensing4 -> waitingState4 [order 1] : [VENT_CMP_DETECT == 1]
  waitingState4 -> ChargingVVIR : after(VentPulseWidth,msec)
  ChargingVVIR -> Sensing4 [order 1] : after(VRP-VentPulseWidth,msec)
  Sensing4 -> PacingVVIR [order 2] : after((RApulseDelay-VentPulseWidth)-(VRP-VentPulseWidth),msec)
  PacingVVIR -> ChargingVVIR : after(VentPulseWidth,msec)
  data: Z_ATR_CTRL output; PACING_REF_PWM output; ATR_GND_CTRL output; PACE_CHARGE_CTRL output; VENT_GND_CTRL output; PACE_GND_CTRL output; Z_VENT_CTRL output; ATR_PACE_CTRL output; VENT_PACE_CTRL output; HIGH constant double =true; LOW constant double =false; pulseDelay input; upperLimit input; AtrialPulseWidth input; atrialAmp input; mode input uint8; VentPulseWidth input; ventAmp input; VRP input; ARP input; Activity_Thres input; Reaction_Time input; Response_Factor input; Recovery_Time input; Atrial_Sense input; Vent_Sense input; ATR_CMP_DETECT input; RApulseDelay input; Max_Sense_Rate input; VENT_CMP_DETECT input
